simulink model "EMPlanner_cs"  (R2020a)
settings: Solver=ode5  StartTime=0.0  StopTime=55  FixedStep=1/1000  RelTol=1e-3
PreLoadFcn:
  | mbxruntime.callbacks.PreLoadFcn(bdroot);
PostLoadFcn:
  | mbxruntime.callbacks.PostLoadFcn(bdroot);
InitFcn:
  | mbxruntime.callbacks.InitFcn(bdroot);
StartFcn:
  | mbxruntime.callbacks.StartFcn(bdroot);
StopFcn:
  | mbxruntime.callbacks.StopFcn(bdroot);
model workspace: external: MAT-File .\EMPlanner_cs_hws.mat (data not in the file)
values from neighbouring files (symbols this model uses):
  c_factor = 43.75    [emplanner_init.m]
  cf = -175016    [emplanner_init.m]
  control_predict_time = 0.01    [emplanner_init.m]
  cr = -130634    [emplanner_init.m]
  dp_col = 4    [emplanner_init.m]
  dp_row = 9    [emplanner_init.m]
  dp_sample_l = 1    [emplanner_init.m]
  dp_sample_s = 15    [emplanner_init.m]
  dp_w_obs = 1e8    (= 100000000)    [emplanner_init.m]
  dp_w_ref = 20    [emplanner_init.m]
  dp_w_smooth_dddl = 10000    [emplanner_init.m]
  dp_w_smooth_ddl = 2000    [emplanner_init.m]
  dp_w_smooth_dl = 300    [emplanner_init.m]
  KD_PID_distance = 0.0    (= 0)    [emplanner_init.m]
  KD_PID_speed = 0    [emplanner_init.m]
  KI_PID_distance = 0.0    (= 0)    [emplanner_init.m]
  KI_PID_speed = 0    [emplanner_init.m]
  KP_PID_distance = 0.5    [emplanner_init.m]
  KP_PID_speed = 1.8    [emplanner_init.m]
  la = 1.265    [emplanner_init.m]
  lb = 2.947-1.265    (= 1.682)    [emplanner_init.m]
  LQR_K1 = k(:,1)'    [emplanner_init.m]
  LQR_K2 = k(:,2)'    [emplanner_init.m]
  LQR_K3 = k(:,3)'    [emplanner_init.m]
  LQR_K4 = k(:,4)'    [emplanner_init.m]
  m = 2020    [emplanner_init.m]
  path_x = [7.7742 8.77358225507 9.77170536558 10.7685522493 11.7641171228 12.7583983581 13.7513958557 14.7431100776 15.7335416918 16.7226914411 17.7105600952 18.6971484329 ... (551 elements, 551x1)]    [test_path.mat]
  path_y = [-207.8202 -207.82020006 -207.820200616 -207.820202023 -207.82020429 -207.820207237 -207.820210603 -207.820214131 -207.82021762 -207.820220941 -207.820224011 -207.820226778 ... (551 elements, 551x1)]    [test_path.mat]
  qp_referenceline_w_length = 2    [emplanner_init.m]
  qp_referenceline_w_ref = 3    [emplanner_init.m]
  qp_referenceline_w_smooth = 1    [emplanner_init.m]
  qp_referenceline_x_lb = -0.2    [emplanner_init.m]
  qp_referenceline_x_ub = 0.2    [emplanner_init.m]
  qp_referenceline_y_lb = -0.2    [emplanner_init.m]
  qp_referenceline_y_ub = 0.2    [emplanner_init.m]
  rack_displacement = [-39.14 , -37.2 , -35.29 , -33.43 , -31.6 , -29.81 , -28.06 , -26.34 , -24.66 ,      -23.01 , -21.38 , -19.79 , -18.23 , -16.69 , -15.18 , -13.7 , -12.23 , -10.8 , -9.38 , -7.98 ,     -6.61 , -5.25 , -3.91 , -2.59 , -1.29 , 0 , 1.27 , 2.54 , 3.78 , 5.02 , 6.24 , 7.46 , 8.66 ,      9.86 , 11.05 , 12.24 , 13.41 , 14.59 , 15.76 , 16.92 , 18.09 , 19.25 , 20.42 , 21.59 , 22.76 ,      23.93 , 25.11 , 26 ...(+26 chars)    [emplanner_init.m]
  right_wheel_ground = [-70 ,-67.2 , -64.4 , -61.6 , -58.8 , -56 , -53.2 , -50.4 , -47.6 , -44.8 , -42 ,      -39.2 , -36.4 , -33.6 , -30.8 , -28 , -25.2 , -22.4 , -19.6 , -16.8 , -14 , -11.2 , -8.4 , -5.6 ,      -2.8 , 0 , 2.8 , 5.6 , 8.4 , 11.2 , 14 , 16.8 , 19.6 , 22.4 , 25.2 , 28 , 30.8 , 33.6 , 36.4 ,      39.2 , 42 , 44.8 , 47.6 , 50.4 , 53.2 , 56 , 58.8 , 61.6 , 64.4 , 67.2 , 70 ]    [emplanner_init.m]
  vx_break_point = zeros(1,5000)    [emplanner_init.m]
undefined symbols (not defined in the file or in its folder): aubr, DiscIntNeverNeededParam, tablebr, vubr, warningInitialVelocity, x0
libraries: simulink x19, PreScanSimulinkLibrary x12, simulink_extras x5, Solver_SF x1
(part 9 of 9)

== matlab function EMPlanner_cs/Audi_A8_Sedan_1/decision&planning module/referenceline provider/MATLAB Function1 ==
  data: x_set_gcs input; match_point_index_set output; y_set_gcs input; path_x_set_gcs input; path_y_set_gcs input; path_heading_set_gcs input; path_kappa_set_gcs input; proj_point_x_set_gcs output; proj_point_y_set_gcs output; proj_point_heading_set_gcs output; proj_point_kappa_set_gcs output
function [match_point_index_set,proj_point_x_set_gcs,proj_point_y_set_gcs,proj_point_heading_set_gcs,...
    proj_point_kappa_set_gcs] = fcn(x_set_gcs,y_set_gcs,path_x_set_gcs,path_y_set_gcs,...
    path_heading_set_gcs,path_kappa_set_gcs)
% 该函数将批量计算点在给定路径下的匹配点编号和投影点信息   
% x_set_gcs,y_set_gcs 输入点信息集合
% path_x_set_gcs,path_y_set_gcs,path_heading_set_gcs,path_kappa_set_gcs 给定路径点信息集合
% match_point_index_set 匹配点编号集合
% proj_point_x_set_gcs,proj_point_y_set_gcs,proj_point_heading_set_gcs,proj_point_kappa_set_gcs 投影点信息集合

% 假设最多有181个点需要投影
n = 181;
% 对输出进行初始化
match_point_index_set = ones(n,1) *nan; 
proj_point_x_set_gcs = ones(n,1) *nan;  proj_point_y_set_gcs = ones(n,1) *nan;
proj_point_heading_set_gcs = ones(n,1) *nan;  proj_point_kappa_set_gcs = ones(n,1) *nan;

% 寻找匹配点时 需要利用上一个周期的结果 因此定义需要利用的静态变量
persistent is_first_run;
persistent pre_match_point_index_set;
persistent pre_path_x_set_gcs; persistent pre_path_y_set_gcs; % 通过上个周期匹配点位矢判断遍历方向
persistent pre_path_heading_set_gcs; persistent pre_path_kappa_set_gcs;
persistent pre_x_set_gcs; persistent pre_y_set_gcs; % 判断相邻帧检测的是否是同一个障碍物

if isempty(is_first_run)
    is_first_run = 0;
    % 首次运行 所有待求点都从给定路径路径第一个点开始找 往前遍历 且距离连续增长上限设为50
    for i = 1:length(x_set_gcs) % 存在的点都在前面 遍历到nan至后面的点都不存在
        if isnan(x_set_gcs(i))
            break;
        end
        start_find_index = 1; forward_stable_backward = 1; increase_count_limit = 50;
        % 计算匹配点编号
        match_point_index = CalMatchPointIndex(x_set_gcs(i),y_set_gcs(i),path_x_set_gcs,...
        path_y_set_gcs,path_heading_set_gcs,path_kappa_set_gcs,start_find_index,...
        increase_count_limit, forward_stable_backward);
        % 计算投影点信息
        [proj_point_x_gcs,proj_point_y_gcs,proj_point_heading_gcs,proj_point_kappa_gcs] = ...
        CalProjPointInfo(x_set_gcs(i),y_set_gcs(i),path_x_set_gcs,path_y_set_gcs,path_heading_set_gcs,...
        path_kappa_set_gcs,match_point_index);
        % 将每个点求解信息添加到集合
        match_point_index_set(i) = match_point_index;
        proj_point_x_set_gcs(i) = proj_point_x_gcs; proj_point_y_set_gcs(i) = proj_point_y_gcs;
        proj_point_heading_set_gcs(i) = proj_point_heading_gcs; 
        proj_point_kappa_set_gcs(i) = proj_point_kappa_gcs;
    end
    % 保存该周期信息 以便下周期使用
    pre_match_point_index_set = match_point_index_set;
    pre_path_x_set_gcs = path_x_set_gcs; pre_path_y_set_gcs = path_y_set_gcs;
    pre_path_heading_set_gcs = path_heading_set_gcs; pre_path_kappa_set_gcs = path_kappa_set_gcs;
    pre_x_set_gcs = x_set_gcs; pre_y_set_gcs = y_set_gcs;
else
    % 需要使用上周期信息
    for i = 1:length(x_set_gcs)
        if isnan(x_set_gcs(i))
            break;
        end
        % 检测相邻帧是否是同一物体求解
        dis = sqrt((x_set_gcs(i)-pre_x_set_gcs(i))^2 + (y_set_gcs(i)-pre_y_set_gcs(i))^2);
        if dis > 10  % 相邻帧(相隔0.1s)同一物体距离不可能这么大
            % 说明相邻帧不是同一物体 上周期该物体已经消失在车辆的检测范围内
            % 把上周期该物体匹配点编号信息清空
            pre_match_point_index_set(i) = nan;
        end
        if isnan(pre_match_point_index_set(i))
            % 说明该物体是第一次寻找匹配点 从头开始寻找 且往前遍历
            start_find_index = 1; forward_stable_backward = 1; increase_count_limit = 50;
        else
            % 说明该物体上周期已经寻找过匹配点  判断开始寻找编号 和遍历方向
            start_find_index = pre_match_point_index_set(i); increase_count_limit = 5;
            % 提取上周期匹配点信息
            pre_match_point_x = pre_path_x_set_gcs(pre_match_point_index_set(i));
            pre_match_point_y = pre_path_y_set_gcs(pre_match_point_index_set(i));
            pre_match_point_heading = pre_path_heading_set_gcs(pre_match_point_index_set(i));
            % 通过该物体上周期匹配点位置到本周期位置向量和上周期匹配点切向量的点乘来判断遍历方向
            vector_preMatch_current = [x_set_gcs(i),y_set_gcs(i)] - [pre_match_point_x, pre_match_point_y];
            vector_tor_preMatch = [cos(pre_match_point_heading), sin(pre_match_point_heading)];
            forward_stable_backward = dot(vector_preMatch_current, vector_tor_preMatch);
        end
        % 计算匹配点编号
        match_point_index = CalMatchPointIndex(x_set_gcs(i),y_set_gcs(i),path_x_set_gcs,...
        path_y_set_gcs,path_heading_set_gcs,path_kappa_set_gcs,start_find_index,...
        increase_count_limit, forward_stable_backward);
        % 计算投影点信息
        [proj_point_x_gcs,proj_point_y_gcs,proj_point_heading_gcs,proj_point_kappa_gcs] = ...
        CalProjPointInfo(x_set_gcs(i),y_set_gcs(i),path_x_set_gcs,path_y_set_gcs,path_heading_set_gcs,...
        path_kappa_set_gcs,match_point_index);
        % 将每个点求解信息添加到集合
        match_point_index_set(i) = match_point_index;
        proj_point_x_set_gcs(i) = proj_point_x_gcs; proj_point_y_set_gcs(i) = proj_point_y_gcs;
        proj_point_heading_set_gcs(i) = proj_point_heading_gcs; 
        proj_point_kappa_set_gcs(i) = proj_point_kappa_gcs;
    end
    % 保存该周期信息 以便下周期使用
    pre_match_point_index_set = match_point_index_set;
    pre_path_x_set_gcs = path_x_set_gcs; pre_path_y_set_gcs = path_y_set_gcs;
    pre_path_heading_set_gcs = path_heading_set_gcs; pre_path_kappa_set_gcs = path_kappa_set_gcs;
    pre_x_set_gcs = x_set_gcs; pre_y_set_gcs = y_set_gcs;
end
end

== matlab function EMPlanner_cs/Audi_A8_Sedan_1/control module2/control main/lateral control LQR/calc lqr K ==
  data: k1 input; k output; k2 input; k3 input; k4 input; vx input
function k  = fcn(k1,k2,k3,k4,vx)
    if abs(vx)<0.1
        k=[0,0,0,0];
    else
       
        k=[k1,k2,k3,k4];
    end
end

== matlab function EMPlanner_cs/Audi_A8_Sedan_1/control module2/control main/lateral control LQR/err_kappa_calculate_module ==
  data: x input; y input; phi input; vx input; vy input; phi_dot input; xr input; yr input; thetar input; kappar input; err output; es output; s_dot output; phi output; projection_point_thetar output
function [err,es,s_dot,phi,projection_point_thetar] = fcn(x,y,phi,vx,vy,phi_dot,xr,yr,thetar,kappar)
    
    tor=[cos(thetar);sin(thetar)];
    nor=[-sin(thetar);cos(thetar)];
    d_err=[x-xr;y-yr];
    ed=nor'*d_err;
    es=tor'*d_err;
    %projection_point_thetar=thetar(dmin);%apollo
    projection_point_thetar=thetar+kappar*es;
    ed_dot=vy*cos(phi-projection_point_thetar)+vx*sin(phi-projection_point_thetar);
    %%%%%%%%%
    ephi=sin(phi-projection_point_thetar);
    %%%%%%%%%
    ss_dot=vx*cos(phi-projection_point_thetar)-vy*sin(phi-projection_point_thetar);
    s_dot=ss_dot/(1-kappar*ed);
    ephi_dot=phi_dot-kappar*s_dot;
    err=[ed;ed_dot;ephi;ephi_dot];
    
    
    
    
    
    
    
    
    
    
    
    


end

== matlab function EMPlanner_cs/Audi_A8_Sedan_1/control module2/control main/lateral control LQR/feed_forword_control ==
  data: vx input; a input; forword_angle output; b input; m input; cf input; cr input; k input; kr input
function forword_angle = fcn(vx,a,b,m,cf,cr,k,kr)
    forword_angle=kr*(a+b-b*k(3)-(m*vx*vx/(a+b))*((b/cf)+(a/cr)*k(3)-(a/cr)));
end

== matlab function EMPlanner_cs/Audi_A8_Sedan_1/control module2/control main/lateral control LQR/feedback_control+feedforword_control ==
  data: k input; angle output; err input; forword_angle input
function angle = fcn(k,err,forword_angle)

    angle=-k*err+forword_angle;
end

== matlab function EMPlanner_cs/Audi_A8_Sedan_1/control module2/control main/lateral control LQR/predict_module ==
  data: x input; pred_x_ctrl output; y input; phi input; vx input; vy input; phi_dot input; ts input; pred_y_ctrl output; pred_yaw_ctrl output; pred_vx_ctrl output; pred_vy_ctrl output; pred_yaw_dot_ctrl output
function [pred_x_ctrl,pred_y_ctrl,pred_yaw_ctrl,pred_vx_ctrl,pred_vy_ctrl,pred_yaw_dot_ctrl] = fcn(x,y,phi,vx,vy,phi_dot,ts)
    pred_x_ctrl=x+vx*ts*cos(phi)-vy*ts*sin(phi);
    pred_y_ctrl=y+vy*ts*cos(phi)+vx*ts*sin(phi);
    pred_yaw_ctrl=phi;
    pred_vx_ctrl=vx;
    pred_vy_ctrl=vy;
    pred_yaw_dot_ctrl=phi_dot;
end

== matlab function EMPlanner_cs/Audi_A8_Sedan_1/control module2/control main/longitudinal control double PID/MATLAB Function1 ==
  data: u input; throttle output; brake output
function [throttle,brake] = fcn(u)
    if u>=0
        throttle=u;
        brake=0;
    else
        throttle=0;
        brake=-u;
    end

== matlab function EMPlanner_cs/Audi_A8_Sedan_1/decision&planning module/EM Planner/calc speed planning start condition ==
  data: plan_start_vx input; plan_start_s_dot output; plan_start_vy input; plan_start_ax input; plan_start_ay input; plan_start_heading input; plan_start_s_dot2 output
function [plan_start_s_dot,plan_start_s_dot2] = fcn(plan_start_vx,plan_start_vy,plan_start_ax,plan_start_ay,plan_start_heading)
% 该函数计算速度规划的初始条件
tor = [cos(plan_start_heading);sin(plan_start_heading)];
v_t = tor'*[plan_start_vx;plan_start_vy];
a_t = tor'*[plan_start_ax;plan_start_ay];
plan_start_s_dot = v_t;
plan_start_s_dot2 = a_t;

== matlab function EMPlanner_cs/Audi_A8_Sedan_1/decision&planning module/EM Planner/simple speed qp planning ==
  data: plan_start_s_dot input; s_init output; plan_start_s_dot2 input; s_end input; recommend_T input; s_dot_init output; s_dot2_init output; relative_time_init output
function [s_init,s_dot_init,s_dot2_init,relative_time_init] = fcn(plan_start_s_dot,plan_start_s_dot2,s_end,recommend_T)
%简单速度二次规划
coder.extrinsic("quadprog")
n = 51;
s_init = zeros(n,1);
s_dot_init = zeros(n,1);
s_dot2_init = zeros(n,1);
relative_time_init = zeros(n,1);

Aeq = zeros(3*n,2*n - 2);
beq = zeros(2*n - 2,1);
lb = ones(3*n,1);
ub = lb;
dt = recommend_T/(n-1);
A_sub =[1,0;
        dt,1;
        (1/3)*dt^2,(1/2)*dt;
        -1,0;
        0,-1;
        (1/6)*dt^2,dt/2];
for i = 1:n - 1
    Aeq(3*i-2:3*i+3,2*i-1:2*i) = A_sub;
end

for i = 1:n
   lb(3*i - 2) = -inf;
   lb(3*i - 1) = 0;
   lb(3*i) = -8;
   ub(3*i - 2) = inf;
   ub(3*i - 1) = 50;
   ub(3*i) = 2;
end
lb(1) = 0;
lb(2) = plan_start_s_dot;
lb(3) = plan_start_s_dot2;
ub(1) = lb(1);
ub(2) = lb(2);
ub(3) = lb(3);
lb(3*n - 2) = s_end;
ub(3*n - 2) = s_end;
A3 = zeros(3*n,3*n);
A4 = zeros(3*n,n - 1);
A4_sub =[0;0;1;0;0;-1];
for i = 1:n - 1
   A3(3*i,3*i) = 1;
   A4(3*i-2:3*i+3,i:i) = A4_sub;
end
A3(3*n,3*n) = 1;
H = A3 + 100*(A4*A4');
H = 2*H;
f = zeros(3*n,1);
X = quadprog(H,f,[],[],Aeq',beq,lb,ub);
for i = 1:n
   s_init(i) = X(3*i - 2);
   s_dot_init(i) = X(3*i - 1);
   s_dot2_init(i) = X(3*i);
   relative_time_init(i) = (i - 1)*dt;
end

== matlab function EMPlanner_cs/Audi_A8_Sedan_1/perception module 自车感知模块/计算出障碍物的绝对位置信息和速度信息 ==
  data: host_x_gcs input; obs_x_set_gcs output; host_y_gcs input; host_heading_gcs input; obs_range_set_sensor input; obs_y_set_gcs output; obs_velocity_set_gcs output; obs_velocity_heading_set_gcs output; obs_theta_set_sensor input; obs_velocity_set_sensor input; obs_velocity_heading_set_sensor input
function [obs_x_set_gcs,obs_y_set_gcs,obs_velocity_set_gcs,obs_velocity_heading_set_gcs] = ...
    fcn(host_x_gcs,host_y_gcs,host_heading_gcs,obs_range_set_sensor,obs_theta_set_sensor,obs_velocity_set_sensor,obs_velocity_heading_set_sensor)
% gcs 全局坐标系   global coordinate system
% 感知模块
% 输入：host_x,host_y,host_heading 自身车辆信息
% obs_range_set_sensor,obs_theta_set_sensor,obs_velocity_set_sensor,obs_velocity_heading_set_sensor 传感器检测到的障碍物信息
% range:障碍物离传感器的直线距离
% theta: 车辆前进方向与障碍物和传感器连线的夹角 顺时针为正 逆时针为负
% velocity:传感器检测到的障碍物的绝对速度
% velocity_heading:障碍物的速度与正北方向的夹角 以北为轴 顺时针旋转为正
% 输出:obs_x_set_gcs,obs_y_set_gcs,obs_velocity_set_gcs,obs_velocity_heading_set_gcs 障碍物在全局坐标下的信息
% 传感器最多识别n个障碍物   n是固定的  即为传感器最多检测障碍物的个数
% 输出初始化
n = length(obs_range_set_sensor);
obs_x_set_gcs = ones(n, 1) * nan;
obs_y_set_gcs = ones(n, 1) * nan;
obs_velocity_set_gcs = ones(n, 1) * nan;
obs_velocity_heading_set_gcs = ones(n, 1) * nan;
% for i = 1:n
%     % 把当前检测到的障碍物信息放进数组 没有检测到的置为nan 
%     % 相当于当前检测到的障碍物都放在数组前面  等到nan为止表示后面的障碍物都不存在
%     if  obs_range_set_sensor(i) ~= 0  %等于0时表示传感器没有检测到该障碍物  无需计算 或者该障碍物不存在
%         % 相邻帧之间障碍物的下标不会改变
%         % 2.16 为传感器到车辆质心的距离
%         obs_x_set_gcs(count) = host_x_gcs + 2.16*cos(host_heading_gcs) + obs_range_set_sensor(i)*cos(host_heading_gcs-obs_theta_set_sensor(i));
%         obs_y_set_gcs(count) = host_y_gcs + 2.16*sin(host_heading_gcs) + obs_range_set_sensor(i)*sin(host_heading_gcs-obs_theta_set_sensor(i));
%         obs_velocity_set_gcs(count) = obs_velocity_set_sensor(i);
%         obs_velocity_heading_set_gcs(count) = pi/2 - obs_velocity_heading_set_sensor(i);
%         count = count + 1;
%     end
% end
for i = 1:n
    % 把当前检测到的障碍物信息放进数组 没有检测到的置为nan 
    % 相当于当前检测到的障碍物都放在数组前面  等到nan为止表示后面的障碍物都不存在
    if  obs_range_set_sensor(i) ~= 0  %等于0时表示传感器没有检测到该障碍物  无需计算 或者该障碍物不存在
        % 相邻帧之间障碍物的下标不会改变
        % 2.16 为传感器到车辆质心的距离
        obs_x_set_gcs(i) = host_x_gcs + 2.16*cos(host_heading_gcs) + obs_range_set_sensor(i)*cos(host_heading_gcs-obs_theta_set_sensor(i));
        obs_y_set_gcs(i) = host_y_gcs + 2.16*sin(host_heading_gcs) + obs_range_set_sensor(i)*sin(host_heading_gcs-obs_theta_set_sensor(i));
        obs_velocity_set_gcs(i) = obs_velocity_set_sensor(i);
        obs_velocity_heading_set_gcs(i) = pi/2 - obs_velocity_heading_set_sensor(i);
    end
end

end

== matlab function EMPlanner_cs/Audi_A8_Sedan_1/decision&planning module/referenceline provider/MATLAB Function2 ==
  data: host_match_point_index input; referenceline_x_init_set_gcs output; path_x_set_gcs input; path_y_set_gcs input; referenceline_y_init_set_gcs output
function [referenceline_x_init_set_gcs, referenceline_y_init_set_gcs] = fun(host_match_point_index, ...
    path_x_set_gcs, path_y_set_gcs)
% 该函数将在给定路径上提取初始参考线
%  host_match_point_index 自车在给定路径上匹配点编号
%  path_x_set_gcs, path_y_set_gcs 给定路径坐标信息
%  referenceline_x_init_set_gcs, referenceline_y_init_set_gcs 初始参考线信息
% 在给定路径上 由匹配点编号往前进方向取150个点  往后退方向取30个点  总共181个点  给定路径一般肯定会多于181个点
% 需要判断 前进方向是否有150个点  或者后退方向是否有30个点
% 从起点着手  一定取得是181个点
if host_match_point_index <= 30
    % 后退方向不够30个点
    start_index = 1; % 从起点开始取
elseif host_match_point_index + 150 > length(path_x_set_gcs)
    % 前进方向不够150个点 则后退方向多取些点
    start_index = length(path_x_set_gcs) - 180;
else
    % 前进和后退方向点的数量均满足要求
    start_index = host_match_point_index - 30;
end

% 在给定路径上提取181个点作为初始参考线 
% referenceline_x_init_set_gcs = path_x_set_gcs(start_index:end_index); %不支持变矩阵
% referenceline_y_init_set_gcs = path_y_set_gcs(start_index:end_index);
referenceline_x_init_set_gcs = path_x_set_gcs(start_index:start_index + 180);
referenceline_y_init_set_gcs = path_y_set_gcs(start_index:start_index + 180);
end
